simulink model "testNmpcPred_sim"  (R2022a)
settings: Solver=FixedStepAuto  StartTime=0.0  StopTime=0.5  FixedStep=0.01  RelTol=1e-3
values from neighbouring files (symbols this model uses):
  N = n+6    [ee_dyn_check.m]    (also in testNmpcPred.m = 12)
  q0 = zeros(N, 1)    [ee_dyn_check.m]    (also in testNmpcPred.m = xTT(seconds(0), :).xk(1:N)')
  q_dot_0 = zeros(N, 1)    [ee_dyn_check.m]    (also in testNmpcPred.m = x_dot_0)
  x_dot_0 = xTT(seconds(0), :).xk(N + 7:2 * N + 6)'    [testNmpcPred.m]
undefined symbols (not defined in the file or in its folder): xee0, xee_dot_0
settings Model: Creator=charl  LastModifiedBy=charl

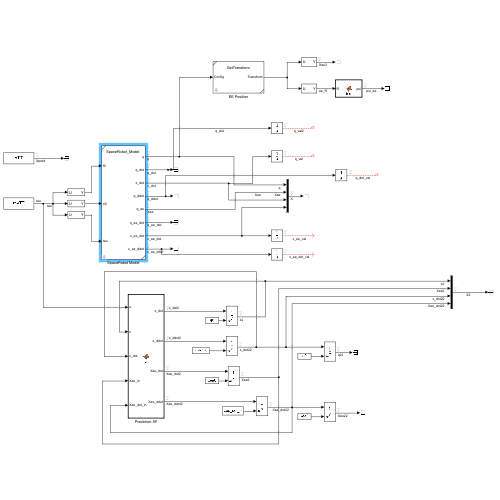
[thumbnail: Simulink's stored preview of the top-level diagram]
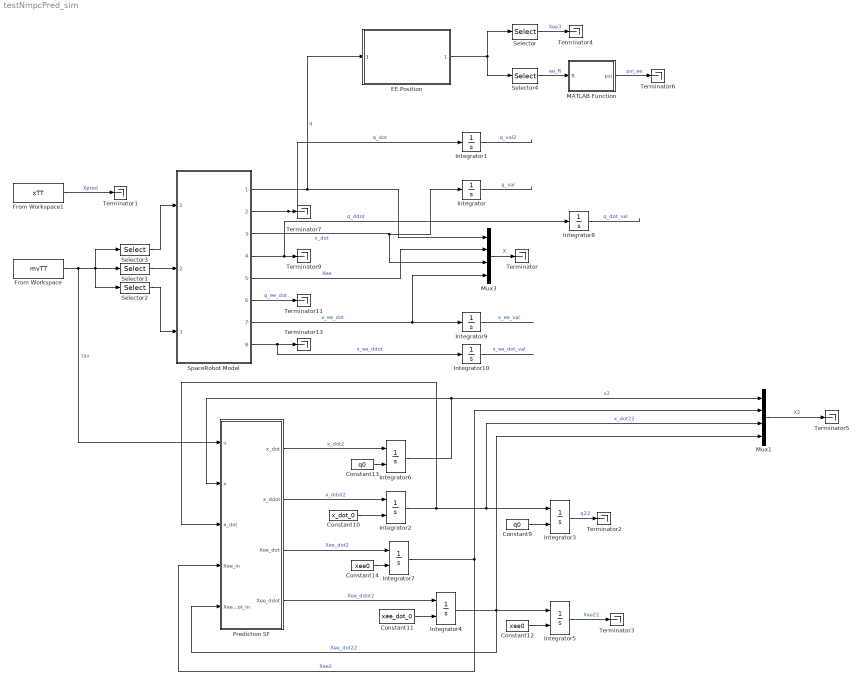
== system testNmpcPred_sim ==
  Constant10 : Constant  Value=x_dot_0
  Constant11 : Constant  Value=xee_dot_0
  Constant12 : Constant  Value=xee0
  Constant13 : Constant  Value=q0
  Constant14 : Constant  Value=xee0
  Constant9 : Constant  Value=q0
  EE Position : Subsystem  ReferencedSubsystem=GetTransform  spaceRobot=sr  sourceBody=endeffector  targetBody=inertial  SimulateUsing=Interpreted execution
  From Workspace : FromWorkspace  VariableName=mvTT
  From Workspace1 : FromWorkspace  VariableName=xTT
  Integrator : Integrator  InitialCondition=q0
  Integrator1 : Integrator  InitialCondition=q0
  Integrator10 : Integrator  InitialCondition=xee_dot_0
  Integrator{2..7} (6 alike) : Integrator  InitialConditionSource=external
  Integrator8 : Integrator  InitialCondition=q_dot_0
  Integrator9 : Integrator  InitialCondition=xee0
  MATLAB Function : MATLAB Function  TreatAsAtomicUnit=on
  Mux1 : Mux
  Mux3 : Mux
  Prediction SF : MATLAB Function  TreatAsAtomicUnit=on
  Selector : Selector  NumberOfDimensions=2  InputPortWidth=[4 4]  IndexOptions=Index vector (dialog),Index vector (dialog)  Indices=[1:3],4  OutputSizes=1,1
  Selector1 : Selector  IndexOptions=Index vector (dialog)  Indices=[4:6]  OutputSizes=1
  Selector2 : Selector  IndexOptions=Index vector (dialog)  Indices=[7:N]  OutputSizes=1
  Selector3 : Selector  IndexOptions=Index vector (dialog)  Indices=[1:3]  OutputSizes=1
  Selector4 : Selector  NumberOfDimensions=2  InputPortWidth=[4 4]  IndexOptions=Index vector (dialog),Index vector (dialog)  Indices=[1:3],[1:3]  OutputSizes=1,1
  SpaceRobot Model : Subsystem  ReferencedSubsystem=SpaceRobot_Model  spaceRobot=sr  jointCstr=off  q_0=q0  q_dot_0=q_dot_0
  Terminator{,1..7,9,11,13} (11 alike) : Terminator
  wires:
  Selector3/1 -> SpaceRobot Model/1
  From Workspace/1 -> Prediction SF/1(u), Selector2/1, Selector1/1, Selector3/1  "tau"
  Selector2/1 -> SpaceRobot Model/3
  Selector1/1 -> SpaceRobot Model/2
  SpaceRobot Model/5 -> Mux3/2  "Xee"
  From Workspace1/1 -> Terminator1/1  "Xpred"
  Constant9/1 -> Integrator3/2
  Integrator6/1 -> Mux1/1, Prediction SF/2(x)  "x2"
  Prediction SF/4(Xee_ddot) -> Integrator4/1  "Xee_ddot2"
  Constant12/1 -> Integrator5/2
  Integrator3/1 -> Terminator2/1  "q22"
  Integrator7/1 -> Prediction SF/4(Xee_in), Mux1/2  "Xee2"
  Constant10/1 -> Integrator2/2
  Integrator2/1 -> Prediction SF/3("x_dot "), Mux1/3, Integrator3/1  "x_dot22"
  Constant13/1 -> Integrator6/2
  Prediction SF/2(x_ddot) -> Integrator2/1  "x_ddot2"
  Prediction SF/3(Xee_dot) -> Integrator7/1  "Xee_dot2"
  Prediction SF/1(x_dot) -> Integrator6/1  "x_dot2"
  Integrator5/1 -> Terminator3/1  "Xee22"
  Constant14/1 -> Integrator7/2
  Integrator4/1 -> Mux1/4, Integrator5/1, Prediction SF/5(Xee_dot_in)  "Xee_dot22"
  Constant11/1 -> Integrator4/2
  Mux1/1 -> Terminator5/1  "X2"
  SpaceRobot Model/3 -> Integrator/1, Mux3/3  "x_dot"
  EE Position/1 -> Selector4/1, Selector/1
  Selector/1 -> Terminator4/1  "Xee3"
  Selector4/1 -> MATLAB Function/1(R)  "ee_R"
  MATLAB Function/1(psi) -> Terminator6/1  "psi_ee"
  Mux3/1 -> Terminator/1  "X"
  SpaceRobot Model/1 -> Mux3/1, EE Position/1  "q"
  SpaceRobot Model/2 -> Integrator1/1, Terminator7/1  "q_dot"
  SpaceRobot Model/4 -> Integrator8/1, Terminator9/1  "q_ddot"
  SpaceRobot Model/6 -> Terminator11/1  "q_ee_dot"
  SpaceRobot Model/7 -> Integrator9/1, Mux3/4  "x_ee_dot"
  SpaceRobot Model/8 -> Integrator10/1, Terminator13/1  "x_ee_ddot"
  Integrator/1 -> ?  "q_val"
  Integrator1/1 -> ?  "q_val2"
  Integrator8/1 -> ?  "q_dot_val"
  Integrator9/1 -> ?  "x_ee_val"
  Integrator10/1 -> ?  "x_ee_dot_val"

== matlab function testNmpcPred_sim/Prediction SF ==
  data: u input; x_dot output; x input; x_ddot output; Xee_dot output; x_dot input; Xee_in input; Xee_dot_in input; Xee_ddot output
function [x_dot, x_ddot, Xee_dot, Xee_ddot] = fcn(u, x, x_dot, Xee_in, Xee_dot_in)

% q_dot(4:6) = omega2euler(q(4:6), q_dot(4:6));
% Xee_dot(4:6) = omega2euler(Xee(4:6), Xee_dot(4:6));

x = [x; Xee_in; x_dot; Xee_dot_in];

% sr_info = SR2_info();
sr_info = SR6_info();


N = sr_info.N;

dx = sr_ee_state_func(x, u, sr_info);

x_dot = dx(1:N);
x_ddot = dx(N+7:2*N+6);

Xee_dot = dx(N+1:N+6);
Xee_ddot = dx(end-5:end);

== matlab function testNmpcPred_sim/MATLAB Function ==
  data: R input; psi output
function psi = fcn(R)

psi = zeros(3, 1);
temp = rotm2eul(R, 'ZYX');
psi(1) = temp(3);
psi(2) = temp(2);
psi(3) = temp(1);
